simulink model "UHDQPSKReceiver"  (R2017b)
settings: Solver=FixedStepDiscrete  StartTime=0.0  StopTime=10.0  RelTol=1e-3
PreLoadFcn:
  | fmRxParams = helperGetFMConfig;
InitFcn:
  | fmRxParams = helperGetFMConfig;
  | 
  | % Check if the radio is configured to receive FM band
  | plutoradioCheckConfig(100e6);
libraries: simulink x1, dspsnks4 x1, commdigbbndpm3 x1, sdrrlib x1
settings Model: Creator=The MathWorks, Inc.  LastModifiedBy=bstac
settings CodeAppCC: StateflowObjectComments=on

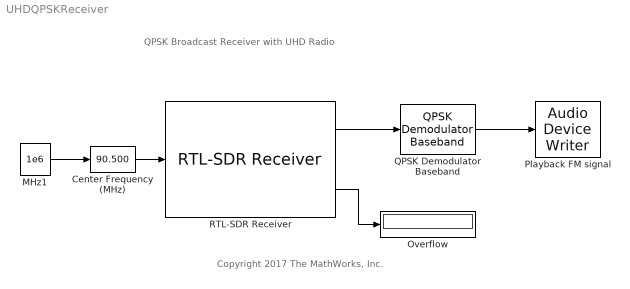
== system UHDQPSKReceiver ==
  note: Copyright 2017 The MathWorks, Inc.
  note: QPSK Broadcast Receiver with UHD Radio
  Center Frequency (MHz) : simulink/Math Operations/Slider Gain  gain=90.500  low=90.3  high=90.7
  MHz1 : Constant  Value=1e6  VectorParams1D=off  SampleTime=fmRxParams.FrontEndSamplesPerFrame/fmRxParams.FrontEndSampleRate  FramePeriod=-1
  Overflow : Display
  Playback FM signal : dspsnks4/Audio Device Writer  Driver=DirectSound  Device=Default  InheritSampleRate=on  SampleRate=44100  BitDepth=16-bit integer  BufferSize=4096  NumBuffers=10  DefaultOutputChannelMapping=on  OutputChannelMapping=1:2  OutputNumUnderrunSamples=off  DriverIdx=1  DeviceWarnFlag=''
  QPSK Demodulator Baseband : commdigbbndpm3/QPSK Demodulator Baseband  OutType=Integer  DecType=Hard decision  VarSource=Dialog  Variance=1  Dec=Gray  Ph=pi/4  outDtype1=int16  outDtype2=Inherit via internal rule  derotateFactorWordLen=16  derotateFactorDataTypeStr=Inherit: Same word length as input  derotateFactorLastDataTypeStr=Inherit: Same word length as input
  RTL-SDR Receiver : sdrrlib/RTL-SDR Receiver  SourceLibraryInfo="This block requires <a href=\"http://www.mathworks.com/hardware-support/rtl-sdr.html\">Communications System Toolbox Support Package for RTL-SDR Radio</a>"  IPAddress=0  CenterFrequencySource=Input port  CenterFrequency=102.5e6  GainSource=AGC  Gain=0  ADCRate=250e3  FrequencyCorrection=0  LostSamplesOutputPort=on  LatencyOutputPort=off  OutputDataType=int16  FrameLength=1024  EnableBurstMode=off  NumFramesInBurst=20  sobjType=sdrr.internal.SDRRTLReceiverSL  dataUDPPort=-1  ctrlUDPPort=-1  subDeviceList=nosubdev  sdrBlockType=SDRBlockTypeSLT.SDRRxBlock  requester=UNUSED_BY_SFCN  sdrExecutionMode=SDRExecutionModeSLT.ExecModeHW  BypassUserLogic=off  DecimatorSelect=DDC decimator  SourceSelect=RF data  SineAmplitude=16000  EnableInternalClock=off  BypassIQBalance=off  IFBandwidth=40e6  ADCRateSource=Dialog  IntermediateFrequency=0  DecimationFactorSource=Dialog  DecimationFactor=512  RFFrequencyIsTunable=logical(1)  SampleTime=(1024)/(250e3)  IFBandwidthSource=Dialog  SineFrequency=30000  BypassDCBlockingFilter=off  IntermediateFrequencySource=Dialog  IQBalanceCoefficients=64  SkipAllHardwareResetAndInitialization=off  EnableIQCalibrationTable=on  CacheIQCalibrationTable=off  EnableOffsetTuning=off  EnableRTLAGC=off  EnableTestMode=off  EnableTunerAGC=on  FrequencyCorrectionSource=Dialog  NumMLBuffers=128  NumUSBBuffers=16  RTLCrystalFrequency=28800000  TunerCrystalFrequency=28800000
      settings: SourceProductName=Communications System Toolbox Support Package for RTL-SDR Radio  SourceProductBaseCode=RTLSDR
  wires:
  RTL-SDR Receiver/2 -> Overflow/1
  QPSK Demodulator Baseband/1 -> Playback FM signal/1
  MHz1/1 -> Center Frequency (MHz)/1
  RTL-SDR Receiver/1 -> QPSK Demodulator Baseband/1
  Center Frequency (MHz)/1 -> RTL-SDR Receiver/1
